simulink model "HoornSimulation_V3"  (R2020b)
settings: Solver=FixedStepAuto  StartTime=0.0  StopTime=100  FixedStep=0.01  RelTol=1e-3
libraries: simulink x4
settings Model: Creator=WANGY17  LastModifiedBy=ASUS
settings DataIOCC: LimitDataPoints=on  SaveFormat=Array  ReturnWorkspaceOutputs=off
settings OptimizationCC: BlockReduction=off  BooleanDataType=off  LifeSpan=inf
settings DebuggingCC: SaveWithParameterizedLinksMsg=none  UnderspecifiedInitializationDetection=Classic  MergeDetectMultiDrivingBlocksExec=none  SignalResolutionControl=TryResolveAllWithWarning  SFUnexpectedBacktrackingDiag=warning  SFNoUnconditionalDefaultTransitionDiag=warning  SFExecutionAtInitializationDiag=none  ArithmeticOperatorsInVariantConditions=warning
settings HardwareCC: ProdBitPerPointer=32  ProdBitPerSizeT=32  ProdBitPerPtrDiffT=32  ProdLargestAtomicFloat=None  ProdIntDivRoundTo=Undefined  ProdEndianess=Unspecified  ProdWordSize=32  ProdHWDeviceType=32-bit Generic  TargetUnknown=on
settings ModelReferenceCC: PropagateSignalLabelsOutOfModel=off
settings SFSimCC: SimUseLocalCustomCode=off  CustomCodeUndefinedFunction=UseInterfaceOnly
settings RTWCC: RTWUseLocalCustomCode=off
settings CodeAppCC: StateflowObjectComments=on
settings GRTTargetCC: TargetLangStandard=C89/C90 (ANSI)
settings ConfigComp: CovMetricSettings=dw  CovSaveCumulativeToWorkspaceVar=on  CovSaveSingleToWorkspaceVar=on  CovExternalEMLEnable=off  CovSFcnEnable=off

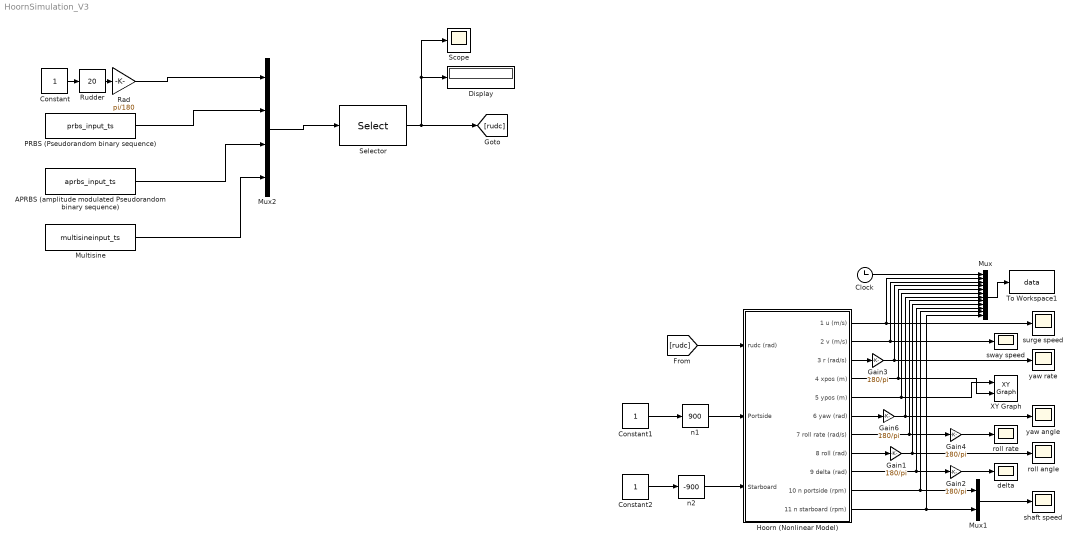
== system HoornSimulation_V3 ==
  APRBS (amplitude modulated Pseudorandom binary sequence) : FromWorkspace  VariableName=aprbs_input_ts
  Clock : Clock
  Constant : Constant
  Constant1 : Constant
  Constant2 : Constant
  Display : Display
  Gain{1..4,6} (5 alike) : Gain  Gain=180/pi
  Hoorn (Nonlinear Model) : Subsystem
  Multisine : FromWorkspace  VariableName=multisineinput_ts
  Mux : Mux  Inputs=12
  Mux1 : Mux  Inputs=2
  Mux2 : Mux
  PRBS (Pseudorandom binary sequence) : FromWorkspace  VariableName=prbs_input_ts
  Rad : Gain  Gain=pi/180  SaturateOnIntegerOverflow=on  OutDataTypeStr=Inherit: Same as input  ParamDataTypeStr=Inherit: Same as input
  Rudder : simulink/Math Operations/Slider Gain  gain=20  low=-30  high=30
  Scope : Scope
  Selector : Selector  InputPortWidth=4  IndexOptions=Index vector (dialog)  Indices=4  OutputSizes=1
  To Workspace1 : ToWorkspace  VariableName=data  SampleTime=-1
      settings: Decimation=2
  XY Graph : simulink/Sinks/XY Graph  xmin=-100  xmax=100  ymin=-100  ymax=100  st=-1
  delta : Scope
  n1 : simulink/Math Operations/Slider Gain  gain=900  low=-1000  high=1000
  n2 : simulink/Math Operations/Slider Gain  gain=-900  low=-1000  high=1000
  roll angle : Scope
  roll rate : Scope
  shaft speed : Scope
  surge speed : Scope
  sway speed : Scope
  yaw angle : Scope
  yaw rate : Scope
  wires:
  Hoorn (Nonlinear Model)/4(4 xpos (m)) -> Mux/5, XY Graph/2
  Hoorn (Nonlinear Model)/5(5 ypos (m)) -> Mux/6, XY Graph/1
  Gain6/1 -> Mux/7, yaw angle/1
  Hoorn (Nonlinear Model)/9(9 delta (rad)) -> Mux/10, Gain2/1
  Gain2/1 -> delta/1
  Hoorn (Nonlinear Model)/8(8 roll (rad)) -> Gain1/1
  Gain1/1 -> Mux/9, roll angle/1
  Hoorn (Nonlinear Model)/7(7 roll rate (rad/s)) -> Mux/8, Gain4/1
  Gain4/1 -> roll rate/1
  Mux/1 -> To Workspace1/1
  Hoorn (Nonlinear Model)/1(1 u (m/s)) -> Mux/2, surge speed/1
  Hoorn (Nonlinear Model)/2(2 v (m/s)) -> Mux/3, sway speed/1
  Hoorn (Nonlinear Model)/3(3 r (rad/s)) -> Gain3/1
  Hoorn (Nonlinear Model)/10(10 n portside (rpm)) -> Mux/11, Mux1/1
  Constant/1 -> Rudder/1
  Rudder/1 -> Rad/1
  Hoorn (Nonlinear Model)/6(6 yaw (rad)) -> Gain6/1
  Gain3/1 -> Mux/4, yaw rate/1
  Constant1/1 -> n1/1
  n1/1 -> Hoorn (Nonlinear Model)/2(Portside)
  Constant2/1 -> n2/1
  n2/1 -> Hoorn (Nonlinear Model)/3(Starboard)
  Hoorn (Nonlinear Model)/11(11 n starboard (rpm)) -> Mux/12, Mux1/2
  Mux1/1 -> shaft speed/1
  Clock/1 -> Mux/1
  Rad/1 -> Mux2/1
  Mux2/1 -> Selector/1
  Selector/1 -> Scope/1, Display/1, [rudc]
  [rudc] -> Hoorn (Nonlinear Model)/1(rudc (rad))
  PRBS (Pseudorandom binary sequence)/1 -> Mux2/2
  APRBS (amplitude modulated Pseudorandom binary sequence)/1 -> Mux2/3
  Multisine/1 -> Mux2/4

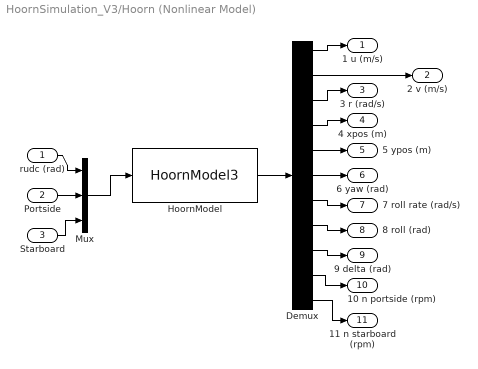
== system HoornSimulation_V3/Hoorn (Nonlinear Model) ==
  rudc (rad) : Inport
  Portside : Inport  Port=2
  Starboard : Inport  Port=3
  Demux : Demux  Outputs=11
  HoornModel : S-Function  FunctionName=HoornModel3  SFunctionDeploymentMode=off  EnableBusSupport=off
  Mux : Mux  Inputs=3
  1 u (m/s) : Outport
  2 v (m/s) : Outport  Port=2
  3 r (rad/s) : Outport  Port=3
  4 xpos (m) : Outport  Port=4
  5 ypos (m) : Outport  Port=5
  6 yaw (rad) : Outport  Port=6
  7 roll rate (rad/s) : Outport  Port=7
  8 roll (rad) : Outport  Port=8
  9 delta (rad) : Outport  Port=9
  10 n portside (rpm) : Outport  Port=10
  11 n starboard (rpm) : Outport  Port=11
  wires:
  Mux/1 -> HoornModel/1
  HoornModel/1 -> Demux/1
  Demux/1 -> 1 u (m/s)/1
  Demux/2 -> 2 v (m/s)/1
  Demux/3 -> 3 r (rad/s)/1
  Demux/4 -> 4 xpos (m)/1
  Demux/5 -> 5 ypos (m)/1
  rudc (rad)/1 -> Mux/1
  Demux/6 -> 6 yaw (rad)/1
  Portside/1 -> Mux/2
  Demux/7 -> 7 roll rate (rad/s)/1
  Demux/8 -> 8 roll (rad)/1
  Demux/9 -> 9 delta (rad)/1
  Demux/10 -> 10 n portside (rpm)/1
  Starboard/1 -> Mux/3
  Demux/11 -> 11 n starboard (rpm)/1
